simulink model "scar"  (R2019a)
settings: Solver=VariableStepAuto  StartTime=0.0  StopTime=5  RelTol=1e-3
values from neighbouring files (symbols this model uses):
  A = [-0.231185976061678;-0.498866089249557;5.84393669821388;3.73021803318506;9.90763303129933]    [rlocus.m]
  B = [4.16554325826943;-0.893946443952200;43.7489661560407;792.115696320530;120.101219035737]    [rlocus.m]
undefined symbols (not defined in the file or in its folder): DiscIntNeverNeededParam
libraries: simulink x1
settings Model: Creator=ray  LastModifiedBy=USER
settings DebuggingCC: AlgebraicLoopMsg=none

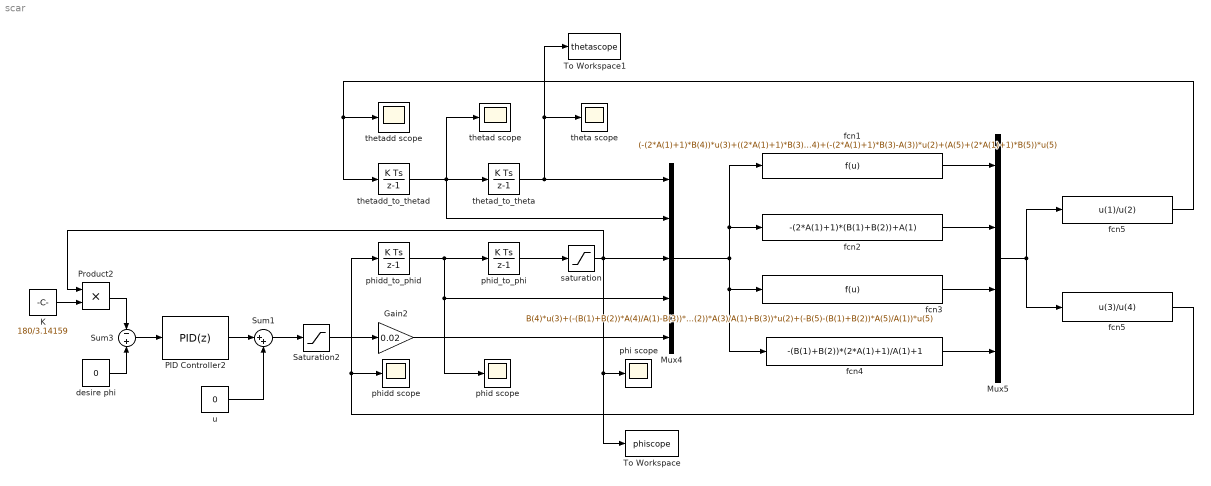
== system scar ==
  Gain2 : Gain  Gain=0.02
  K : Constant  Value=180/3.14159  SampleTime=0.01
  Mux4 : Mux  Inputs=5
  Mux5 : Mux
  PID Controller2 : simulink/Continuous/PID Controller  Controller=PID  Form=Parallel  TimeDomain=Discrete-time  SampleTime=0.001  IntegratorMethod=Forward Euler  FilterMethod=Forward Euler  ControllerParametersSource=internal  P=10  I=500  D=0.01  UseFilter=on  N=100  TunerSelectOption=Transfer Function Based (PID Tuner App)  InitialConditionSource=internal  InitialConditionForIntegrator=0  InitialConditionForFilter=0  DifferentiatorICPrevScaledInput=0  ExternalReset=none  TrackingMode=off  Kt=1  LimitOutput=off  UpperSaturationLimit=inf  LowerSaturationLimit=-inf  LinearizeAsGain=on  AntiWindupMode=none  Kb=1  POutMin=[]  POutMax=[]  IOutMin=[]  IOutMax=[]  DOutMin=[]  DOutMax=[]  NOutMin=[]  NOutMax=[]  SumOutMin=[]  SumOutMax=[]  SaturationOutMin=[]  SaturationOutMax=[]  PParamMin=[]  PParamMax=[]  IParamMin=[]  IParamMax=[]  DParamMin=[]  DParamMax=[]  NParamMin=[]  NParamMax=[]  KbParamMin=[]  KbParamMax=[]  KtParamMin=[]  KtParamMax=[]  KbOutMin=[]  KbOutMax=[]  KtOutMin=[]  KtOutMax=[]  IntegratorOutMin=[]  IntegratorOutMax=[]  FilterOutMin=[]  FilterOutMax=[]  SumI1OutMin=[]  SumI1OutMax=[]  SumI2OutMin=[]  SumI2OutMax=[]  SumI3OutMin=[]  SumI3OutMax=[]  SumI4OutMin=[]  SumI4OutMax=[]  SumDOutMin=[]  SumDOutMax=[]  DifferentiatorOutMin=[]  DifferentiatorOutMax=[]  FilterDiffOutCoefMin=[]  FilterDiffOutCoefMax=[]  ReciprocalOutMin=[]  ReciprocalOutMax=[]  SumDenOutMin=[]  SumDenOutMax=[]  SumNumOutMin=[]  SumNumOutMax=[]  DivideOutMin=[]  DivideOutMax=[]  IntegratorContinuousStateAttributes=''  IntegratorStateMustResolveToSignalObject=off  IntegratorRTWStateStorageClass=Auto  FilterContinuousStateAttributes=''  FilterStateMustResolveToSignalObject=off  FilterRTWStateStorageClass=Auto  ParallelPVariant=InternalParameters  IdealPVariant=Disabled  IVariant=InternalParameters  DVariant=InternalParameters  IntegratorVariant=Discrete  SatVariant=Disabled  AWVariant=Passthrough  PCopyVariant=Disabled  TRVariant=Disabled  FdbkBlocksVariant=Forward  IdealPFdbkVariant=Disabled  SatFdbkVariant=Disabled  DerivativeFilterVariant=ForwardEulerFilter  NVariant=InternalParameters  NCopyVariant=Disabled  FilterICVariant=InternalICsFilter  IntegratorICVariant=InternalICs  ExternalResetVariant=Disabled  TRSumVariant=Passthrough  SumFdbkVariant=Disabled  SumVariant=Sum_PID
  Product2 : Product
  Saturation2 : Saturate  UpperLimit=255  LowerLimit=-255
  Sum1 : Sum  Inputs=|++
  Sum3 : Sum  Inputs=-+
  To Workspace : ToWorkspace  VariableName=phiscope  SaveFormat=Timeseries  SampleTime=-1
  To Workspace1 : ToWorkspace  VariableName=thetascope  SaveFormat=Timeseries  SampleTime=-1
  desire phi : Constant  Value=0  SampleTime=0.01
  fcn1 : Fcn  Expr=(-(2*A(1)+1)*B(4))*u(3)+((2*A(1)+1)*B(3)+A(4))*u(4)+(-(2*A(1)+1)*B(3)-A(3))*u(2)+(A(5)+(2*A(1)+1)*B(5))*u(5)
  fcn2 : Fcn  Expr=-(2*A(1)+1)*(B(1)+B(2))+A(1)
  fcn3 : Fcn  Expr=B(4)*u(3)+(-(B(1)+B(2))*A(4)/A(1)-B(3))*u(4)+((B(1)+B(2))*A(3)/A(1)+B(3))*u(2)+(-B(5)-(B(1)+B(2))*A(5)/A(1))*u(5)
  fcn4 : Fcn  Expr=-(B(1)+B(2))*(2*A(1)+1)/A(1)+1
  fcn5 : Fcn  Expr=u(3)/u(4)
  "fcn5 " : Fcn  Expr=u(1)/u(2)
  phi scope : Scope
  phid scope : Scope
  "phid_to_phi " : DiscreteIntegrator  SampleTime=0.01  ICPrevOutput=DiscIntNeverNeededParam  ICPrevScaledInput=DiscIntNeverNeededParam
  phidd scope : Scope
  phidd_to_phid : DiscreteIntegrator  SampleTime=0.01  ICPrevOutput=DiscIntNeverNeededParam  ICPrevScaledInput=DiscIntNeverNeededParam
  saturation : Saturate  UpperLimit=1.57  LowerLimit=-1.57
  "theta scope " : Scope
  thetad scope : Scope
  thetad_to_theta : DiscreteIntegrator  SampleTime=0.01  ICPrevOutput=DiscIntNeverNeededParam  ICPrevScaledInput=DiscIntNeverNeededParam
  thetadd scope : Scope
  thetadd_to_thetad : DiscreteIntegrator  SampleTime=0.01  ICPrevOutput=DiscIntNeverNeededParam  ICPrevScaledInput=DiscIntNeverNeededParam
  u : Constant  Value=0  SampleTime=0.01
  wires:
  Mux5/1 -> fcn5/1, "fcn5 "/1
  Mux4/1 -> fcn1/1, fcn2/1, fcn4/1, fcn3/1
  saturation/1 -> To Workspace/1, phi scope/1, Product2/1, Mux4/3
  Gain2/1 -> Mux4/5
  Saturation2/1 -> Gain2/1
  fcn3/1 -> Mux5/3
  "phid_to_phi "/1 -> saturation/1
  thetadd_to_thetad/1 -> thetad_to_theta/1, Mux4/2, thetad scope/1
  fcn2/1 -> Mux5/2
  fcn1/1 -> Mux5/1
  phidd_to_phid/1 -> "phid_to_phi "/1, phid scope/1, Mux4/4
  fcn4/1 -> Mux5/4
  Sum1/1 -> Saturation2/1
  fcn5/1 -> phidd_to_phid/1, phidd scope/1
  thetad_to_theta/1 -> Mux4/1, To Workspace1/1, "theta scope "/1
  u/1 -> Sum1/2
  "fcn5 "/1 -> thetadd scope/1, thetadd_to_thetad/1
  PID Controller2/1 -> Sum1/1
  Sum3/1 -> PID Controller2/1
  desire phi/1 -> Sum3/2
  K/1 -> Product2/2
  Product2/1 -> Sum3/1
